simulink library "INT_RmtAPP_ChkSig"  (R2016b)
settings: Solver=VariableStepAuto  StartTime=0.0  StopTime=10.0  RelTol=1e-3
settings Model: Creator=bianxuyin  LastModifiedBy=bianxuyin

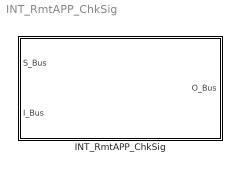
== system INT_RmtAPP_ChkSig ==
  INT_RmtAPP_ChkSig : Subsystem

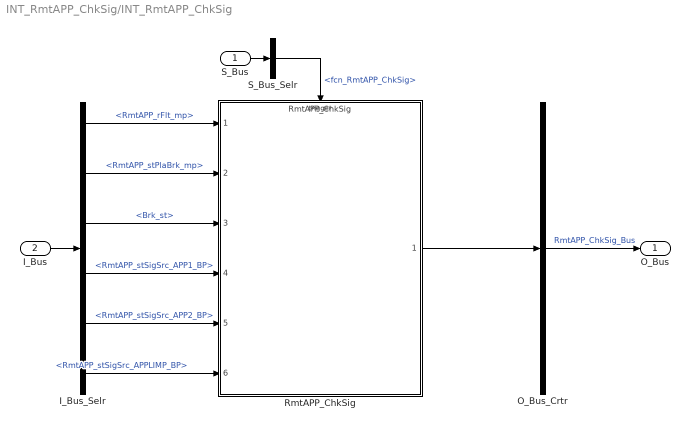
== system INT_RmtAPP_ChkSig/INT_RmtAPP_ChkSig ==
  S_Bus : Inport
  I_Bus : Inport  Port=2
  I_Bus_Selr : BusSelector  OutputSignals=RmtAPP_rFlt_mp,RmtAPP_stPlaBrk_mp,Brk_st,RmtAPP_stSigSrc_APP1_BP,RmtAPP_stSigSrc_APP2_BP,RmtAPP_stSigSrc_APPLIMP_BP
  O_Bus_Crtr : BusCreator  Inputs=1
  RmtAPP_ChkSig : ModelReference  ModelNameDialog=RmtAPP_ChkSig  SimulationMode=Normal  ModelReferenceVersion=1.15  TriggerPortName=function  TriggerPortTriggerType=function-call  TriggerPortStatesWhenEnabling=held
  S_Bus_Selr : BusSelector  OutputSignals=fcn_RmtAPP_ChkSig
  O_Bus : Outport
  wires:
  S_Bus_Selr/1 -> RmtAPP_ChkSig/Trigger  "<fcn_RmtAPP_ChkSig>"
  S_Bus/1 -> S_Bus_Selr/1
  I_Bus/1 -> I_Bus_Selr/1
  I_Bus_Selr/1 -> RmtAPP_ChkSig/1  "<RmtAPP_rFlt_mp>"
  I_Bus_Selr/2 -> RmtAPP_ChkSig/2  "<RmtAPP_stPlaBrk_mp>"
  I_Bus_Selr/3 -> RmtAPP_ChkSig/3  "<Brk_st>"
  I_Bus_Selr/4 -> RmtAPP_ChkSig/4  "<RmtAPP_stSigSrc_APP1_BP>"
  I_Bus_Selr/5 -> RmtAPP_ChkSig/5  "<RmtAPP_stSigSrc_APP2_BP>"
  I_Bus_Selr/6 -> RmtAPP_ChkSig/6  "<RmtAPP_stSigSrc_APPLIMP_BP>"
  O_Bus_Crtr/1 -> O_Bus/1  "RmtAPP_ChkSig_Bus"
  RmtAPP_ChkSig/1 -> O_Bus_Crtr/1
